simulink model "Dyn_Nonlinear_four"  (R2021a)
settings: Solver=VariableStepAuto  StartTime=0.0  StopTime=10  FixedStep=0.048  MaxStep=0.048  RelTol=1e-5
(part 1 of 7)
settings Model: Creator=zahra  LastModifiedBy=Dell 5520
settings SolverCC: AlgebraicLoopSolver=TrustRegion
settings DataIOCC: ReturnWorkspaceOutputs=off
settings DebuggingCC: ArithmeticOperatorsInVariantConditions=warning
settings SFSimCC: CustomCodeUndefinedFunction=UseInterfaceOnly
settings CodeAppCC: StateflowObjectComments=on

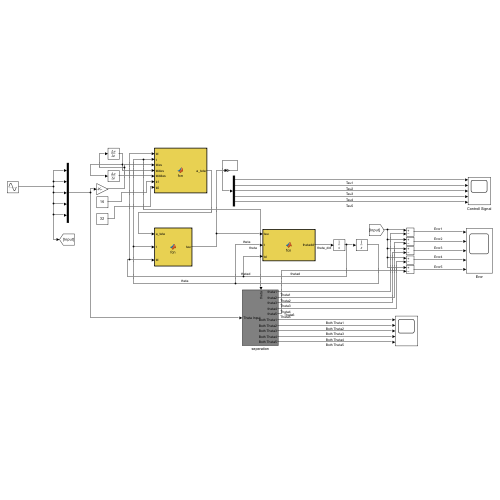
[thumbnail: Simulink's stored preview of the top-level diagram]
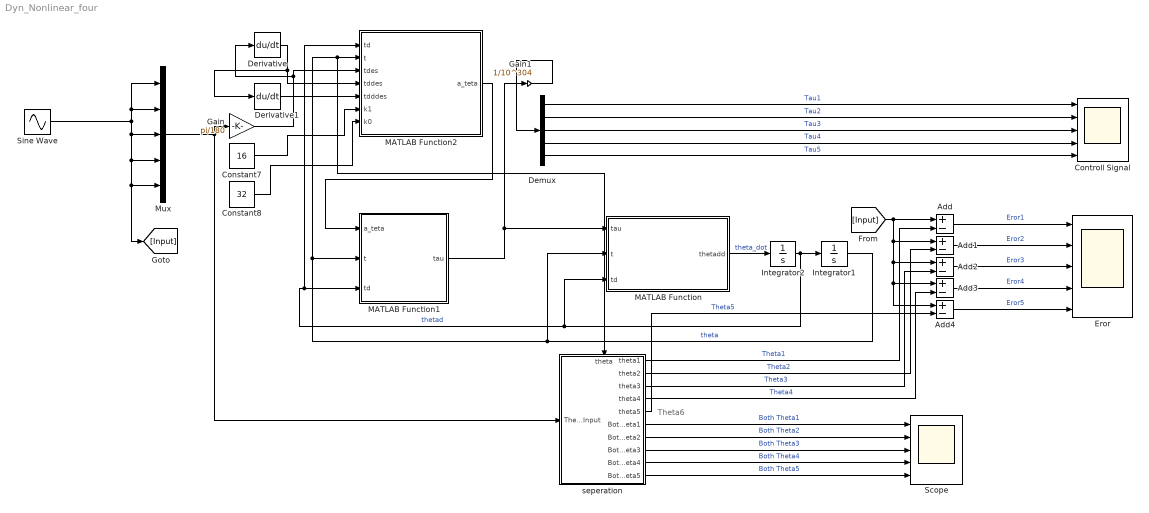
== system Dyn_Nonlinear_four ==
  note: Theta6
  Add{,1..4} (5 alike) : Sum  Inputs=+-
  Constant7 : Constant  Value=16
  Constant8 : Constant  Value=32
  Controll Signal : Scope  NumInputPorts=5
  Demux : Demux  Outputs=5
  Derivative : Derivative
  Derivative1 : Derivative
  Eror : Scope  NumInputPorts=5
  Gain : Gain  Gain=pi/180
  Gain1 : Gain  Gain=1/10^304
  Integrator1 : Integrator  InitialCondition=[0;0;0;0;0]
  Integrator2 : Integrator  InitialCondition=[0;0;0;0;0]
  MATLAB Function : MATLAB Function  TreatAsAtomicUnit=on
  MATLAB Function1 : MATLAB Function  TreatAsAtomicUnit=on
  MATLAB Function2 : MATLAB Function  TreatAsAtomicUnit=on
  Mux : Mux  Inputs=5
  Scope : Scope  NumInputPorts=5
  Sine Wave : Sin  SampleTime=0
  seperation : Subsystem
      settings: PortSchema="{\"entries\":[{\"content\":{\"sides\":[{\"content\":{\"connectorIds\":[\"In1\"]},\"type\":\"ConnectorPlacement.EquallySpacedRectSide\",\"uuid\":\"117984fd-d3d6-4145-babf-48c13158da12\"},{\"content\":{\"connectorIds\":[\"Out1\",\"Out2\",\"Out3\",\"Out4\",\"Out5\",\"Out6\",\"Out7\",\"Out8\",\"Out9\",\"Out10\"],\"side\":\"RIGHT\"},\"type\":\"ConnectorPlacement.EquallySpacedRectSide\",\"uuid\":\"5922d531-a812-4762-9837-e12cfcbe2b47\"},{\"content\":{\"connectorIds\":[\"In2\"],\"side\":\"TOP\"},\"type\":\"ConnectorPlacement.EquallySpacedRectSide\",\"uuid\":\"698f3307-05bd-42ee-8fdc-8fa637aa5a4a\"},{\"content\":{\"connectorIds\":[],\"side\":\"HIDDEN\"},\"type\":\"ConnectorPlacement.EquallySpacedRectSide\",\"uuid\":\"cdbd4c97-0f0a-4dfe-9d96-04d42d36c789\"}]},\"type\":\"ConnectorPlacement.EquallySpacedConnector\",\"uuid\":\"afea5cc0-dec2-4c18-a646-40882511f7cf\"}],\"packageUris\":[\"http://schema.mathworks.com/mf0/Connector/R2020b\"],\"version\":\"1.0\"}"
  wires:
  MATLAB Function/1(thetadd) -> Integrator2/1  "theta_dot"
  Integrator1/1 -> MATLAB Function/2(t), seperation/2(theta), MATLAB Function2/2(t), MATLAB Function1/2(t)  "theta"
  Integrator2/1 -> Integrator1/1, MATLAB Function1/3(td), MATLAB Function2/1(td), MATLAB Function/3(td)  "thetad"
  seperation/1(theta1) -> Add/2  "Theta1"
  seperation/2(theta2) -> Add1/2  "Theta2"
  seperation/3(theta3) -> Add2/2  "Theta3"
  seperation/4(theta4) -> Add3/2  "Theta4"
  seperation/5(theta5) -> Add4/2  "Theta5"
  MATLAB Function1/1(tau) -> Gain1/1, MATLAB Function/1(tau)
  Mux/1 -> Gain/1, seperation/1(Theta Input)
  Constant7/1 -> MATLAB Function2/6(k1)
  Constant8/1 -> MATLAB Function2/7(k0)
  Derivative/1 -> Derivative1/1, MATLAB Function2/4(tddes)
  Derivative1/1 -> MATLAB Function2/5(tdddes)
  MATLAB Function2/1(a_teta) -> MATLAB Function1/1(a_teta)
  Sine Wave/1 -> Mux/3, [Input], Mux/5, Mux/4, Mux/1, Mux/2
  Demux/2 -> Controll Signal/2  "Tau2"
  Demux/1 -> Controll Signal/1  "Tau1"
  Demux/5 -> Controll Signal/5  "Tau5"
  Demux/4 -> Controll Signal/4  "Tau4"
  Demux/3 -> Controll Signal/3  "Tau3"
  Add4/1 -> Eror/5  "Eror5"
  Add1/1 -> Eror/2  "Eror2"
  Add3/1 -> Eror/4  "Eror4"
  Add/1 -> Eror/1  "Eror1"
  Add2/1 -> Eror/3  "Eror3"
  [Input] -> Add4/1, Add3/1, Add2/1, Add1/1, Add/1
  seperation/6(Both Theta1) -> Scope/1  "Both Theta1"
  seperation/7(Both Theta2) -> Scope/2  "Both Theta2"
  seperation/8(Both Theta3) -> Scope/3  "Both Theta3"
  seperation/9(Both Theta4) -> Scope/4  "Both Theta4"
  seperation/10(Both Theta5) -> Scope/5  "Both Theta5"
  Gain/1 -> Derivative/1, MATLAB Function2/3(tdes)
  Gain1/1 -> Demux/1

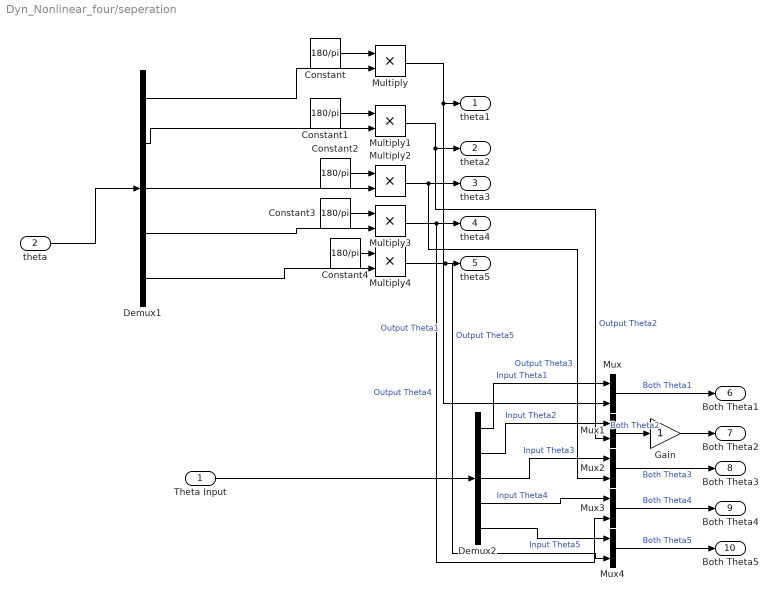
== system Dyn_Nonlinear_four/seperation ==
  Theta Input : Inport
  theta : Inport  Port=2
  Constant{,1..4} (5 alike) : Constant  Value=180/pi
  Demux1 : Demux  Outputs=5
  Demux2 : Demux  Outputs=5
  Gain : Gain
  Multiply{,1..4} (5 alike) : Product
  Mux{,1..4} (5 alike) : Mux  Inputs=2
  theta1 : Outport
  theta2 : Outport  Port=2
  theta3 : Outport  Port=3
  theta4 : Outport  Port=4
  theta5 : Outport  Port=5
  Both Theta1 : Outport  Port=6
  Both Theta2 : Outport  Port=7
  Both Theta3 : Outport  Port=8
  Both Theta4 : Outport  Port=9
  Both Theta5 : Outport  Port=10
  wires:
  theta/1 -> Demux1/1
  Constant/1 -> Multiply/1
  Demux1/1 -> Multiply/2
  Demux1/2 -> Multiply1/2
  Constant1/1 -> Multiply1/1
  Constant2/1 -> Multiply2/1
  Demux1/3 -> Multiply2/2
  Demux1/4 -> Multiply3/2
  Constant3/1 -> Multiply3/1
  Demux1/5 -> Multiply4/2
  Constant4/1 -> Multiply4/1
  Multiply4/1 -> Mux4/2, theta5/1  "Output Theta5"
  Multiply3/1 -> Mux3/2, theta4/1  "Output Theta4"
  Multiply2/1 -> Mux2/2, theta3/1  "Output Theta3"
  Multiply1/1 -> Mux1/2, theta2/1  "Output Theta2"
  Multiply/1 -> Mux/2, theta1/1  "Output Theta1"
  Theta Input/1 -> Demux2/1
  Mux/1 -> Both Theta1/1  "Both Theta1"
  Demux2/2 -> Mux1/1  "Input Theta2"
  Demux2/3 -> Mux2/1  "Input Theta3"
  Demux2/4 -> Mux3/1  "Input Theta4"
  Demux2/5 -> Mux4/1  "Input Theta5"
  Mux1/1 -> Gain/1  "Both Theta2"
  Mux2/1 -> Both Theta3/1  "Both Theta3"
  Mux3/1 -> Both Theta4/1  "Both Theta4"
  Mux4/1 -> Both Theta5/1  "Both Theta5"
  Demux2/1 -> Mux/1  "Input Theta1"
  Gain/1 -> Both Theta2/1

== matlab function Dyn_Nonlinear_four/MATLAB Function2 ==
  data: a_teta output; td input; t input; tdes input; tddes input; tdddes input; k1 input; k0 input
function a_teta = fcn(td,t,tdes,tddes,tdddes,k1,k0)
a_teta= tdddes+k1*(tddes-td)+k0*(tdes-t);

return;
